simulink library "SEN_SUN"  (Simulink 10.2)
settings: Solver=VariableStepAuto  StartTime=0.0  StopTime=10.0  RelTol=1e-3
undefined symbols (not defined in the file): SEN_SUN_par
libraries: LIB_ROT x2, simulink x1
settings Model: Creator=dbell44  LastModifiedBy=dbell44

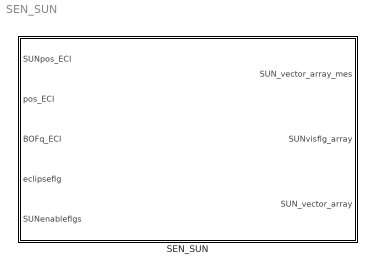
== system SEN_SUN ==
  SEN_SUN : Subsystem

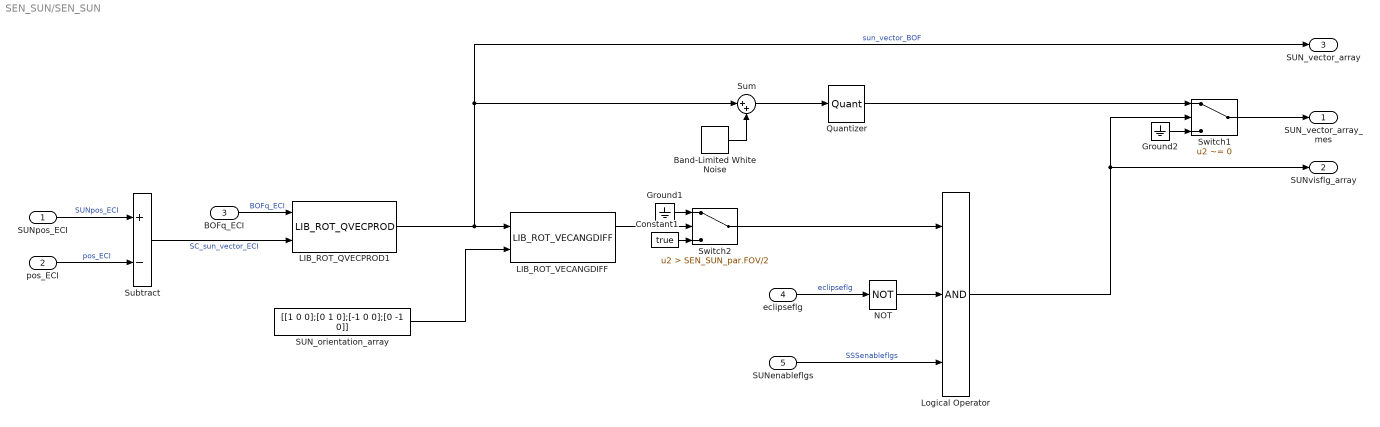
== system SEN_SUN/SEN_SUN ==
  SUNpos_ECI : Inport
  pos_ECI : Inport  Port=2
  BOFq_ECI : Inport  Port=3
  eclipseflg : Inport  Port=4
  SUNenableflgs : Inport  Port=5
  Band-Limited White Noise : simulink/Sources/Band-Limited White Noise  Cov=SEN_SUN_par.noise_power  Ts=1/SEN_SUN_par.sample_rate  seed=randi([1 243453])
  Constant1 : Constant  Value=true
  Ground1 : Ground
  Ground2 : Ground
  LIB_ROT_QVECPROD1 : LIB_ROT/LIB_ROT_QVECPROD
  LIB_ROT_VECANGDIFF : LIB_ROT/LIB_ROT_VECANGDIFF  zero_tol=0
  Logical Operator : Logic  Inputs=3  AllPortsSameDT=off  OutDataTypeStr=boolean
  NOT : Logic  Operator=NOT  IconShape=distinctive  AllPortsSameDT=off  OutDataTypeStr=boolean
  Quantizer : Quantizer  QuantizationInterval=SEN_SUN_par.sensitivity  LinearizeAsGain=off
  SUN_orientation_array : Constant  Value=[[1 0 0];[0 1 0];[-1 0 0];[0 -1 0]]
  Subtract : Sum  Inputs=+-
  Sum : Sum  Inputs=|++
  Switch1 : Switch  Criteria=u2 ~= 0
  Switch2 : Switch  Criteria=u2 > Threshold  Threshold=SEN_SUN_par.FOV/2
  SUN_vector_array_mes : Outport  VectorParamsAs1DForOutWhenUnconnected=off
  SUNvisflg_array : Outport  Port=2  VectorParamsAs1DForOutWhenUnconnected=off
  SUN_vector_array : Outport  Port=3  VectorParamsAs1DForOutWhenUnconnected=off
  wires:
  pos_ECI/1 -> Subtract/2  "pos_ECI"
  SUNpos_ECI/1 -> Subtract/1  "SUNpos_ECI"
  Subtract/1 -> LIB_ROT_QVECPROD1/2  "SC_sun_vector_ECI"
  BOFq_ECI/1 -> LIB_ROT_QVECPROD1/1  "BOFq_ECI"
  LIB_ROT_QVECPROD1/1 -> SUN_vector_array/1, Sum/1, LIB_ROT_VECANGDIFF/1  "sun_vector_BOF"
  SUN_orientation_array/1 -> LIB_ROT_VECANGDIFF/2
  eclipseflg/1 -> NOT/1  "eclipseflg"
  SUNenableflgs/1 -> Logical Operator/3  "SSSenableflgs"
  NOT/1 -> Logical Operator/2
  Band-Limited White Noise/1 -> Sum/2
  Sum/1 -> Quantizer/1
  LIB_ROT_VECANGDIFF/1 -> Switch2/2
  Switch2/1 -> Logical Operator/1
  Ground1/1 -> Switch2/1
  Constant1/1 -> Switch2/3
  Quantizer/1 -> Switch1/1
  Ground2/1 -> Switch1/3
  Logical Operator/1 -> Switch1/2, SUNvisflg_array/1
  Switch1/1 -> SUN_vector_array_mes/1
